simulink model "sim09"  (R2012b)
settings: Solver=ode45  StartTime=0.0  StopTime=20  RelTol=1e-3
undefined symbols (not defined in the file): magnitude
settings Model: Creator=Administrator  LastModifiedBy=Administrator

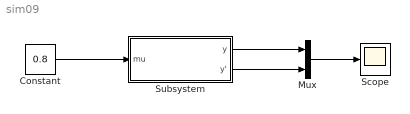
== system sim09 ==
  Constant : Constant  Value=0.8
  Mux : Mux  Inputs=2
  Scope : Scope
  Subsystem : Subsystem
  wires:
  Mux/1 -> Scope/1
  Constant/1 -> Subsystem/1(mu)
  Subsystem/1(y) -> Mux/1
  Subsystem/2(y') -> Mux/2

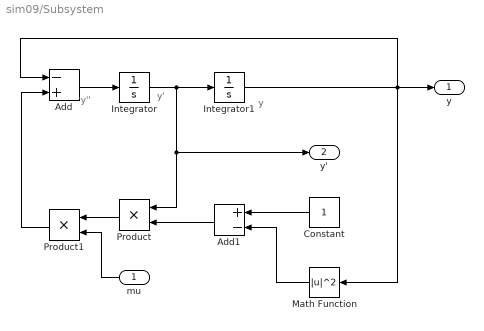
== system sim09/Subsystem ==
  note: y
  note: y'
  note: y''
  mu : Inport
  Add : Sum  Inputs=-+
  Add1 : Sum  Inputs=+-
  Constant : Constant
  Integrator : Integrator  InitialCondition=-2
  Integrator1 : Integrator  InitialCondition=4
  Math Function : Math  Operator=magnitude^2  SaturateOnIntegerOverflow=on
  Product : Product  RndMeth=Zero
  Product1 : Product  RndMeth=Zero
  y : Outport
  y' : Outport  Port=2
  wires:
  Add/1 -> Integrator/1
  Integrator/1 -> Product/1, y'/1, Integrator1/1
  Constant/1 -> Add1/1
  Math Function/1 -> Add1/2
  Add1/1 -> Product/2
  Product/1 -> Product1/1
  Product1/1 -> Add/2
  Integrator1/1 -> Math Function/1, Add/1, y/1
  mu/1 -> Product1/2
